simulink model "Previous_version_Sim_framework"  (R2024a)
settings: Solver=VariableStepAuto  StartTime=0.0  StopTime=10.0  RelTol=1e-3
undefined symbols (not defined in the file or in its folder): DiscIntNeverNeededParam
libraries: aerolibatmos2 x1
settings Model: Creator=nicom  LastModifiedBy=nicom

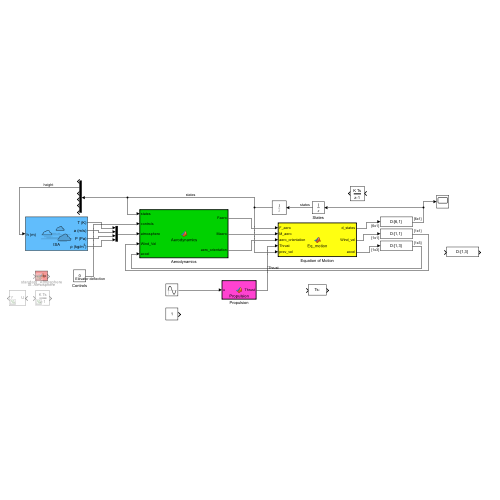
[thumbnail: Simulink's stored preview of the top-level diagram]
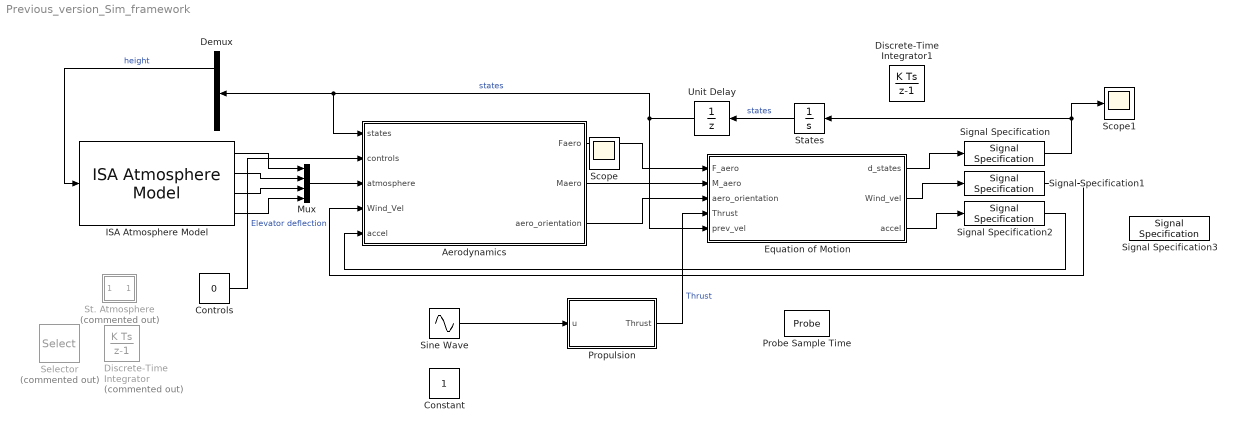
== system Previous_version_Sim_framework ==
  Aerodynamics : MATLAB Function  TreatAsAtomicUnit=on
  Constant : Constant
  Controls : Constant  Value=0
  Demux : Demux  Outputs=6
  Discrete-Time Integrator : DiscreteIntegrator  Commented=on  SampleTime=-1  ICPrevOutput=DiscIntNeverNeededParam  ICPrevScaledInput=DiscIntNeverNeededParam
  Discrete-Time Integrator1 : DiscreteIntegrator  SampleTime=0.001  ICPrevOutput=DiscIntNeverNeededParam  ICPrevScaledInput=DiscIntNeverNeededParam
  Equation of Motion : MATLAB Function  TreatAsAtomicUnit=on
  ISA Atmosphere Model : aerolibatmos2/ISA Atmosphere Model  useExtended=off  action=Warning  custom=off  viscosityOut=off  g=9.80665  gamma=1.4  R=287.0531  L=0.0065  h_trop=11000  h_strat=20000  rho0=1.225  P0=101325  T0=288.15  h0=0  S=110.4  Tref=273.15  muref=1.716e-5
  Mux : Mux
  Probe Sample Time : Probe  ProbeWidth=off  ProbeComplexSignal=off
  Propulsion : MATLAB Function  TreatAsAtomicUnit=on
  Scope1 : Scope
  Selector : Selector  Commented=on  NumberOfDimensions=6  InputPortWidth=3  IndexOptions=Index vector (dialog),Index vector (dialog),Index vector (dialog),Index vector (dialog),Index vector (dialog),Index vector (dialog)  Indices=[1 3],1,1,1,1,1  OutputSizes=1,1,1,1,1,1
  Signal Specification : SignalSpecification  Dimensions=[6,1]
  Signal Specification1 : SignalSpecification  Dimensions=[1,1]
  Signal Specification2 : SignalSpecification  Dimensions=[1,3]
  Signal Specification3 : SignalSpecification  Dimensions=[1,3]
  Sine Wave : Sin  SampleTime=0
  St. Atmosphere : MATLAB Function  Commented=on  TreatAsAtomicUnit=on
  States : Integrator
  Unit Delay : UnitDelay  SampleTime=0.001  HasFrameUpgradeWarning=on
  Scope : Scope
  wires:
  Controls/1 -> Aerodynamics/2(controls)  "Elevator deflection"
  Aerodynamics/1(Faero) -> Equation of Motion/1(F_aero)
  Aerodynamics/2(Maero) -> Equation of Motion/2(M_aero)
  Sine Wave/1 -> Propulsion/1(u)
  Propulsion/1(Thrust) -> Equation of Motion/4(Thrust)  "Thrust"
  Aerodynamics/3(aero_orientation) -> Equation of Motion/3(aero_orientation)
  Unit Delay/1 -> Aerodynamics/1(states), Demux/1, Equation of Motion/5(prev_vel)  "states"
  ISA Atmosphere Model/1 -> Mux/1
  ISA Atmosphere Model/2 -> Mux/2
  ISA Atmosphere Model/3 -> Mux/3
  ISA Atmosphere Model/4 -> Mux/4
  Mux/1 -> Aerodynamics/3(atmosphere)
  Equation of Motion/1(d_states) -> Signal Specification/1
  Signal Specification/1 -> Scope1/1, States/1
  Equation of Motion/2(Wind_vel) -> Signal Specification1/1
  Signal Specification1/1 -> Aerodynamics/4(Wind_Vel)
  Equation of Motion/3(accel) -> Signal Specification2/1
  Signal Specification2/1 -> Aerodynamics/5(accel)
  Demux/2 -> ISA Atmosphere Model/1  "height"
  States/1 -> Unit Delay/1  "states"

== matlab function Previous_version_Sim_framework/St. Atmosphere ==
  data: Atmosphere output; states input
function Atmosphere  = standard_Atmosphere(states)

% states = [x1,x2,x3,   x4,x5,x6, x4_dot, x5_dot, x6_dot];
%          [x  y  Theta Vx Vy q]
% eq_motion = [x1dot,x2dot,x3dot,x4dot,x5dot,x6dot];
%           [Vx    
g = 9.807;


alt = states(2);

[T,a,P,rho,nu,mu] = atmosisa(alt);

Atmosphere = [T,a,P,rho,nu,mu,alt];

% y = states(2);
% alt = y

function [T, a, P, rho, nu, mu] = atmosisa(h,nameValueArg)
%  ATMOSISA Use International Standard Atmosphere Model.
%   [T, A, P, RHO, NU, MU] = ATMOSISA(H) and
%   [T, A, P, RHO, NU, MU] = ATMOSISA(H, 'extended', false) implement the
%   mathematical representation of the International Standard Atmosphere values
%   for ambient temperature, pressure, density, speed of sound, kinematic
%   viscosity, and dynamic viscosity for the input geopotential altitude between
%   the sea level and the tropopause. Density and speed of sound are calculated
%   using a perfect gas relationship.
%
%   [T, A, P, RHO, NU, MU] = ATMOSISA(H, 'extended', true) implements the
%   mathematical representation of the International Standard Atmosphere values
%   for ambient temperature, pressure, density, speed of sound, kinematic
%   viscosity, and dynamic viscosity for the input geopotential altitude between
%   -5000 meters and the mesopause. Density and speed of sound are calculated
%   using a perfect gas relationship.
%
%   Inputs:
%   H         : Numeric array of M-by-N values of geopotential heights in meters.
%
%   Name-Value Pair Arguments:
%   'EXTENDED': Flag to set the upper and lower limits for the input altitude. 
%               When 'extended' is set to false (default), output values are held 
%               for input altitudes below 0 m and above 20000 m (tropopause).
%               When 'extended' is set to true, output values are held for input
%               altitudes below -5000 m and above 84852 m (mesopause).
%   'ACTION'  : A string to determine action for out-of-range input for the 
%               extended (true) model. Specify if out-of-range input invokes a 
%               'warning', 'error', or 'none' (no action). The default is 'warning'.
%
%   Outputs:
%   T         : Numeric array of M-by-N values of temperatures in kelvin.
%   A         : Numeric array of M-by-N values of speed of sound in meters per second.
%   P         : Numeric array of M-by-N values of air pressures in pascals.
%   RHO       : Numeric array of M-by-N values of air densities in kilograms per meter cubed.
%   NU        : Numeric array of M-by-N values of kinematic viscosities in meters squared per
%               second.
%   MU        : Numeric array of M-by-N values of dynamic viscosities in Newton second per 
%               meters squared.
%
%   Limitation:
%   Set upper and lower limits for geopotential altitudes using the 'extended'
%   name-value pair argument.
%
%   If the 'extended' flag is set to false (default), below the geopotential
%   altitude of 0 meters and above the geopotential altitude of the tropopause
%   at 20000 m, the output values are held.
%   If the 'extended' flag is set to true, the implementation is limited to the
%   geopotential altitude of -5000 meters (minimum) and the mesopause at
%   84852 m (maximum).  If the action input is 'error', an input geopotential
%   height outside these limits results in error. If the action input is 'warning'
%   or 'none', the outputs are held at the limits.
%
%   Examples:
%
%   Calculate the International Standard Atmosphere at 1000 meters:
%      [T, a, P, rho, nu, mu] = atmosisa(1000)
%
%   Calculate the International Standard Atmosphere at 1000, 11000, 20000,
%   and 35000 meters using the extended model:
%      [T, a, P, rho, nu, mu] = atmosisa([1000 11000 20000 35000], 'extended', true)
%
%   See also ATMOSCIRA, ATMOSCOESA, ATMOSLAPSE, ATMOSNONSTD.

%   Copyright 2000-2023 The MathWorks, Inc.

%   Reference:  U.S. Standard Atmosphere, 1976, U.S. Government Printing
%   Office, Washington, D.C.


arguments
    h {mustBeNumeric, mustBeReal}
    nameValueArg.extended (1,1) matlab.lang.OnOffSwitchState = false
    nameValueArg.action Aero.internal.datatype.Action = 'warning'
end

action = nameValueArg.action;
useExtended = nameValueArg.extended; % flag to determine the model

g0 = 9.80665;
gamma = 1.4;
beta = 1.458e-6;
S = 110.4;

switch(useExtended)
    case false
        R = 287.0531; % Gas constant value from the initial implementation
        [T, a, P, rho] = atmoslapse(h, g0, gamma, R, 0.0065, 11000, 20000, ...
            1.225, 101325, 288.15 );

    case true
        T = zeros(size(h));
        P = T;

        L = [-0.0065 0 0.001 0.0028 0 -0.0028 -0.002]; % lapse rate for the 8 atmosphere layers
        Hb = [0 11000 20000 32000 47000 51000 71000 84852]; % 8 atmosphere layers
        T0 = [288.1500  216.6500  216.6500  228.6500  270.6500  270.6500  214.6500...
            186.9460]; % base temperature of each layer
        P0 = [101325 22632.0405969347 5474.8776606600 868.0158377494 110.9057845539...
            66.9385353730 3.9563927546 0.3733803710]; % base pressure of each layer
        rho0 = 1.225; % sea level density

        R = P0(1)/(rho0*T0(1)); % Gas constant calculated from sea-level values

        % Handle action for height checking
        handleaction(h, action);

        %Outside the limits of -5000 meters and 84852 meters, the output values are held constant 
        h(h<-5000.0) = -5000.0;
        h(h>84852.0) = 84852.0;

        T(h==0) = T0(1);
        P(h==0) = P0(1);

        hvals = h;
        htmp = h<0;
        if any(htmp, 'all')
            hvals(htmp) = 0;
            T(htmp) = T0(1) + L(1)*(h(htmp)-Hb(1));
            theta = T(htmp)./T0(1);
            P(htmp) = P0(1)*theta.^(-g0/(L(1)*R));
        end

        for HbInd = 1: length(Hb)-1
            if ~any(hvals) %to break the loop if all elements in h have been evaluated
                break;
            end

            htmp = h>Hb(HbInd) & h<=Hb(HbInd+1);

            if any(htmp,'all')

                if L(HbInd)==0
                    T(htmp) = T0(HbInd);
                    P(htmp) = P0(HbInd)*exp((-g0*(h(htmp)-Hb(HbInd)))./(R*T(htmp)));

                else
                    T(htmp) = T0(HbInd) + L(HbInd)*(h(htmp)-Hb(HbInd));
                    theta = T(htmp)./T0(HbInd);
                    P(htmp) = P0(HbInd)*theta.^(-g0/(L(HbInd)*R));

                end
                hvals(htmp) = 0;
            end
        end

        rho = P./(R*T);
        a = sqrt(gamma*R*T);
end

mu = beta*(T.^1.5)./(T+S);
nu = mu./rho;

    function handleaction(h, action)
        switch action
            case "None"
                % no checking of height
            case "Warning"
                if (any(h < -5000.0, "all") || any(h > 84852.0, "all"))
                    warning(message('aero:atmosisa:outsideLimitsWarn'));
                end
            case "Error"
                idx = find(h < -5000.0 | h > 84852.0, 1);
                if ~isempty(idx)
                    error(message('aero:atmosisa:outsideLimitsErr', idx, string(h(idx))));
                end
        end
    end

end
end

== matlab function Previous_version_Sim_framework/Equation of Motion ==
  data: d_states output; F_aero input; M_aero input; aero_orientation input; Thrust input; Wind_vel output; accel output; prev_vel input
function [d_states,Wind_vel,accel] = Eq_motion(F_aero,M_aero,aero_orientation, Thrust,prev_vel)

time_step = 0.001;

% prev

prev_vel1 = prev_vel(4);
prev_vel2 = prev_vel(5);
prev_vel3 = prev_vel(6);


%Acceleration
% x4dot = 1/m*(L*sin(eta) - D*cos(eta) + Lt*sin(gamma) + T*cos(x3) - Nm*mu - N);
% x5dot = 1/m*(L*cos(eta) - D*sin(eta) + Lt*cos(gamma) - T*sin(x3) + W - Nm - Nt);
% x6dot = 1/J * (M + L*xA*cos(alpha) - Lt*xt*cos(alphat) + Nm*alpha - Nt*b);
% L = 1/2 * rho * S * CL * VR2
% D = 1/2 * 

% x1 = states(1); % (x)
% x2 = states(2); % (y)
% x3 = states(3); % (theta)
% x4 = states(4); % (Vx)
% x5 = states(5); % (Vy)
% x6 = states(6); % (q)
% x4_dot = states(7); % (Ax)
% x5_dot = states(8); % (Ay)
% x6_dot = states(9); % (q dot)


% x = x + x4*t + (1/2)at²

% Given Constants
m = 300; %kg
J = 33.03; %kg*m^2



% aero_orientation = [alpha,eta,theta];
alpha = aero_orientation(1);
eta = aero_orientation(2);
theta = aero_orientation(3);
gamma = aero_orientation(4);
alpha_t = aero_orientation(5);

x3 = theta;


T = Thrust;

% Vr = sqrt((x4 + ax)^2 + (x5 + ay)^2); 


% Faero = [L, D, LT]; 
% Maero = M; 
L = F_aero(1); 
D = F_aero(2); 
Lt= F_aero(3); 
M = M_aero(1); 

%Modeling as on ground so 0 normal force
Nm = 0;
Nt = 0;
mu = 0.05; % Rolling Friction Coefficient, assumption of 0.05
W = 300; %kgf
xA = 1.1; %m, Doubtful of this value but maybe is fine
xt = 3.26;
a = 0; % distance of main landing gear to cg
b = 0; % distance of tail landing geat to cg

x4_dot = 1/m*(L*sin(eta) - D*cos(eta) + Lt*sin(gamma) + T*cos(x3) - Nm*mu - Nt*mu);
x5_dot = 1/m*(-L*cos(eta) - D*sin(eta) + Lt*cos(gamma) - T*sin(x3) + W - Nm - Nt);
x6_dot = 1/J * (M + L*xA*cos(alpha) - Lt*xt*cos(alpha_t) + Nm*a - Nt*b);

x4 = x4_dot*time_step + prev_vel1;
x5 = x5_dot*time_step + prev_vel2;
x6 = x6_dot*time_step + prev_vel3;

vel = [x4,x5,x6];

% eq_motion = [x1dot,x2dot,x3dot,x4dot,x5dot,x6dot];

d_states = zeros(6, 1);

% states = [x1,x2,x3,x4,x5,x6,x4_dot,x5_dot,x6_dot];

d_states = [x4,x5,x6,x4_dot,x5_dot,x6_dot]';

% deriv_states = [x4,x5,x6,x4_dot,x5_dot,x6_dot];

accel = [x4_dot,x5_dot,x6_dot];

Wind_vel = 0; % for now
% x4dot    = 

% states = [x1,x2,x3,x4,x5,x6,x4_dot,x5_dot,x6_dot];

== matlab function Previous_version_Sim_framework/Aerodynamics ==
  data: states input; Faero output; controls input; Maero output; atmosphere input; Wind_Vel input; aero_orientation output; accel input
function [Faero, Maero, aero_orientation] = Aerodynamics(states,controls, atmosphere, Wind_Vel,accel)


% states = [x1,x2,x3,x4,x5,x6,x4_dot,x5_dot,x6_dot]

% controls = [delta_elev]
% Atmosphere = [T,a,P,rho,nu,mu,alt];


% Given constants
CD0 = 0.02; 
e = 0.80; 
AR = 7; 
k = 1/(AR*pi*e); 
ST = 1; %m^2
S = 4.74; %m^2
x_t = 3.26;
c_bar = 5; % CHANGE LATER

delta = controls(1);

rho = atmosphere(4);

x1 = states(1); % (x)
x2 = states(2); % (y)
x3 = states(3); % (theta)
x4 = states(4); % (Vx)
x5 = states(5); % (Vy)
x6 = states(6); % (q)

% x4_dot = states(7); % (Ax)
% x5_dot = states(8); % (Ay)
% x6_dot = states(9); % (q dot)
x4_dot = accel(1); % (Ax)
x5_dot = accel(2); % (Ay)
x6_dot = accel(3); % (q dot)

ax = - x4_dot; % Questionable negative here !!!
ay = - x5_dot;
theta = x3;

% Rotation speed in flight
Vr = sqrt((x4 + ax)^2 + (x5 + ay)^2); 

% Flight Path Angle
sineta = ((x5+ay)/Vr);
coseta = ((x4+ax)/Vr);
eta = atan(sineta/coseta);

alpha = theta + eta;

ux = 0; % FIND ACTUAL VALUES FOR THESE
uy = 0;

p = x6 * x_t;
w = alpha * 0.4032*Vr;

V_TT = (x4 + ux)*cos(x3) - (x5 + uy)*sin(x3);
V_NT = (x4 + ux)*sin(x3) + (x5 + uy)*cos(x3) + p-w;
V_RT = sqrt(((x4+ux)^2 + (x5+uy)^2) + (2*(x4+ux)*sin(x3) + 2*(x5+uy)*sin(x3) + p-w) * (p-w));

sin_alpha_t = V_NT/V_RT;
cos_alpha_t = V_TT/V_RT;

alpha_t = atan(sin_alpha_t/cos_alpha_t);

gamma = alpha_t-theta;

[CL] = CL_calc(alpha); 
[CLT] = CLT_calc(alpha_t, delta); 
[CD] = CD_calc(alpha, CD0, k); 
[CM] = CM_calc(alpha); 

V_RT = sqrt((x4 + ux) ^2 + (x5 + uy)^2 + (2*(x4 + ux)*sin(x3) + 2*(x5 +uy)*sin(x3) + p - w) * (p-w)); 

L = 0.5 * rho * S * CL * Vr^2; 
LT = 0.5 * rho * ST * CLT * V_RT^2;
D = 0.5 * rho * S * CD * Vr^2; 
M = 0.5 * rho * S * c_bar * CM * Vr^2; 

Faero = [L, D, LT]; 
Maero = M; 

aero_orientation = [alpha,eta,theta,gamma,alpha_t];
states = [x1+0.01,x2+0.01,x3+0.01,x4+0.01,x5+0.01,x6+0.01]';
end 


function [CL] = CL_calc(alpha)
CL = alpha * 2* pi; 
end 

function [CLT] = CLT_calc(alpha_t, delta)
CLt = alpha_t * 2* pi; 
CLT = CLt * delta; 
end 

function [CD] = CD_calc(alpha, CD0, k)
[CL] = CL_calc(alpha); 
CD = CD0 + k * CL^2; 
end 

function [CM] = CM_calc(alpha)
CM = - alpha * 2* pi; 
end

== matlab function Previous_version_Sim_framework/Propulsion ==
  data: u input; Thrust output
function Thrust = Propulsion(u)

Thrust = u;
